simulink model "PS84OL"  (Simulink 8.2)
settings: Solver=ode45  StartTime=0.0  StopTime=10.0  RelTol=1e-3
values from neighbouring files (symbols this model uses):
  filter_order = 3    [PS8_4.m]
  P_den = [1 2 0]    [PS8_4.m]
  P_num = [1 -a]    [PS8_4.m]
  W2 = r    (= 0.0001)    [PS8_4.m]    (also in PS_8_4.m)
  W3 = r    (= 0.0001)    [PS8_4.m]
  W4 = r    (= 0.0001)    [PS8_4.m]
libraries: dsparch4 x1
settings Model: Creator=Yili  LastModifiedBy=MQ
settings DataIOCC: SignalLoggingSaveFormat=Dataset
settings OptimizationCC: ExpressionDepthLimit=128
settings DebuggingCC: FcnCallInpInsideContextMsg=EnableAllAsError  StateNameClashWarn=none
settings GRTTargetCC: CombineOutputUpdateFcns=on  GRTInterface=off

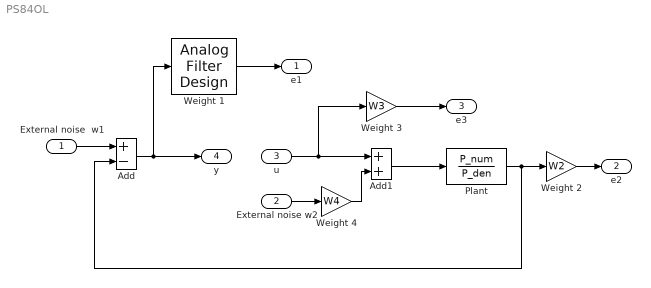
== system PS84OL ==
  External noise  w1 : Inport
  External noise w2 : Inport  Port=2
  u : Inport  Port=3
  Add : Sum  Inputs=+-
  Add1 : Sum
  Plant : TransferFcn  Numerator=P_num  Denominator=P_den
  Weight 1 : dsparch4/Analog Filter Design  method=Butterworth  filttype=Lowpass  N=filter_order  Wlo=cut_off_freq  Whi=80  Rp=2  Rs=40
  Weight 2 : Gain  Gain=W2
  Weight 3 : Gain  Gain=W3
  Weight 4 : Gain  Gain=W4
  e1 : Outport
  e2 : Outport  Port=2
  e3 : Outport  Port=3
  y : Outport  Port=4
  wires:
  External noise  w1/1 -> Add/1
  u/1 -> Add1/1, Weight 3/1
  Add/1 -> Weight 1/1, y/1
  Weight 2/1 -> e2/1
  Weight 3/1 -> e3/1
  Plant/1 -> Add/2, Weight 2/1
  Add1/1 -> Plant/1
  External noise w2/1 -> Weight 4/1
  Weight 4/1 -> Add1/2
  Weight 1/1 -> e1/1
